simulink model "Fig416"  (R2014b)
settings: Solver=FixedStepDiscrete  StartTime=0.0  StopTime=.005  FixedStep=1.25e-6  RelTol=1e-3
libraries: commsrccod2 x4
settings Model: Creator=Dennis Silage  LastModifiedBy=Silage
settings DataIOCC: SignalLoggingSaveFormat=ModelDataLogs
settings OptimizationCC: ExpressionDepthLimit=2147483647  InitFltsAndDblsToZero=on
settings DebuggingCC: UnderspecifiedInitializationDetection=Classic  MergeDetectMultiDrivingBlocksExec=none  FcnCallInpInsideContextMsg=UseLocalSettings  StateNameClashWarn=warning
settings GRTTargetCC: CombineOutputUpdateFcns=off  GRTInterface=on

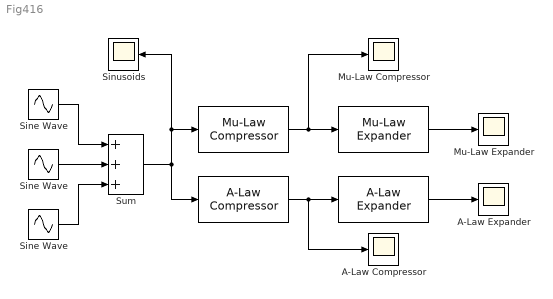
== system Fig416 ==
  " " : commsrccod2/Mu-Law Compressor  mu=255  V=1.5
  "  " : commsrccod2/Mu-Law Expander  mu=255  V=1.5
  "   " : commsrccod2/A-Law Compressor  A=87.6  V=1.5
  "    " : commsrccod2/A-Law Expander  A=87.6  V=1.5
  " Sine Wave " : Sin  Amplitude=0.2  Frequency=5000*pi  SampleTime=1.25e-6
  A-Law Compressor : Scope
      settings: SaveName=ScopeData3
  A-Law Expander : Scope
      settings: SaveName=ScopeData4
  Mu-Law Compressor : Scope
  Mu-Law Expander : Scope
      settings: SaveName=ScopeData2
  Sine Wave : Sin  Frequency=1000*pi  SampleTime=1.25e-6
  "Sine Wave " : Sin  Amplitude=0.5  Frequency=3000*pi  SampleTime=1.25e-6
  Sinusoids : Scope
      settings: YMin=-1.5  YMax=1.5  SaveName=ScopeData5
  Sum : Sum  Inputs=+++
  wires:
  " "/1 -> "  "/1, Mu-Law Compressor/1
  "  "/1 -> Mu-Law Expander/1
  "   "/1 -> "    "/1, A-Law Compressor/1
  "    "/1 -> A-Law Expander/1
  "Sine Wave "/1 -> Sum/2
  " Sine Wave "/1 -> Sum/3
  Sine Wave/1 -> Sum/1
  Sum/1 -> "   "/1, " "/1, Sinusoids/1
